simulink model "TrafficLightNegotiationWithV2XTestBench"  (R2024b)
settings: Solver=ode23tb  StartTime=0.0  StopTime=scenario.StopTime  FixedStep=0.1  RelTol=1e-8  EnableMultiTasking=on
PostLoadFcn:
  | helperSLTrafficLightNegotiationWithV2XSetup
values from neighbouring files (symbols this model uses):
  actorsClassID = [[profiles.ActorID]' [profiles.ClassID]' [profiles.Length]' [profiles.Width]']    [helperSLTrafficLightNegotiationWithV2XSetup.m]
  intersectionInfo = evalin('base', 'intersectionInfo')    [HelperTLNwithV2XVisualization.m]
  posSelector = [ 1, 0, 0, 0, 0, 0, 0, 0, 0; 0, 0, 0, 1, 0, 0, 0, 0, 0]    [helperSLTrafficLightNegotiationWithV2XSetup.m]
  referencePathInfo = helperEgoRefPathCreator(scenario, egoVehicle.ActorID)    [helperSLTrafficLightNegotiationWithV2XSetup.m]
  sceneOrigin = [42.2995, -83.6990, 0]    [helperSLTrafficLightNegotiationWithV2XSetup.m]
undefined symbols (not defined in the file or in its folder): M, N, Ts, v_set
libraries: drivingscenarioandsensors x2, simulink x1, drivinglib x1
CloseFcn:
  | helperSLTrafficLightNegotiationWithV2XCleanUp
settings Model: SnapshotBufferSize=50  SnapshotInterval=1  Creator=The MathWorks, Inc.  LastModifiedBy=Pranith
settings SolverCC: ZeroCrossAlgorithm=Adaptive  AlgebraicLoopSolver=TrustRegion  PositivePriorityOrder=on  AutoInsertRateTranBlk=on  InsertRTBMode=Always  DecoupledContinuousIntegration=on  MinimalZcImpactIntegration=on  MaxZcPerStep=1
settings DataIOCC: SaveOutput=off  SaveTime=off  ReturnWorkspaceOutputs=off
settings OptimizationCC: ReuseModelBlockBuffer=off
settings DebuggingCC: MaskedZcDiagnostic=none  IgnoredZcDiagnostic=none  ParameterPrecisionLossMsg=none  UnconnectedInputMsg=warning  UnconnectedOutputMsg=warning  UnconnectedLineMsg=warning  PregeneratedLibrarySubsystemCodeDiagnostic=none  SubsystemReferenceDiagnosticForUnitTest=warning  ArithmeticOperatorsInVariantConditions=warning
settings HardwareCC: ProdLongLongMode=on
settings ModelReferenceCC: EnableRefExpFcnMdlSchedulingChecks=on
settings SFSimCC: SimUseLocalCustomCode=off
settings RTWCC: GenerateReport=on  RTWUseLocalCustomCode=off  LaunchReport=on  GPUComputeCapability=3.5  DLArmComputeVersion=19.05
settings ConfigComp: CovScope=ReferencedModels  CovIncludeTopModel=off

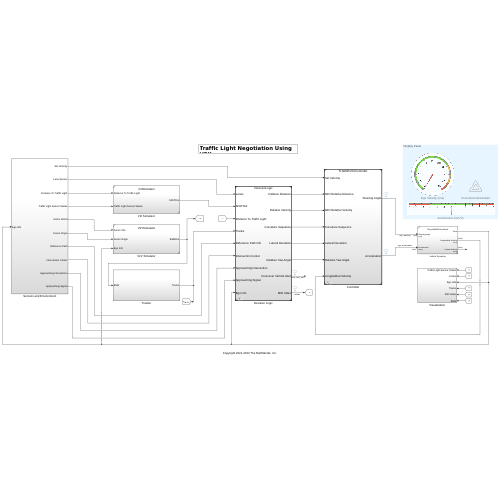
[thumbnail: Simulink's stored preview of the top-level diagram]
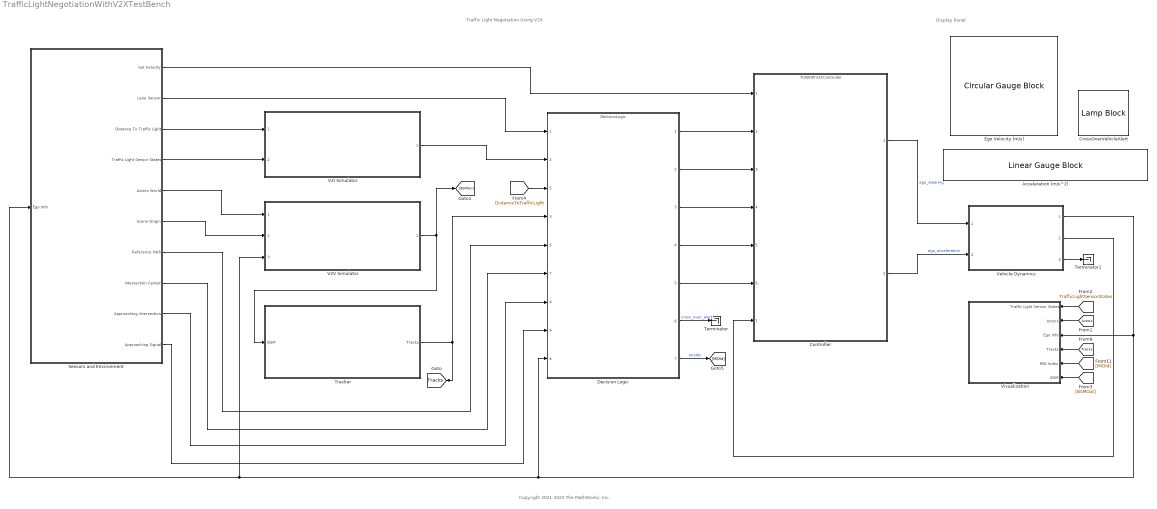
== system TrafficLightNegotiationWithV2XTestBench ==
  note: Traffic Light Negotiation Using V2X
  note: Display Panel
  note: Copyright 2021-2023 The MathWorks, Inc.
  Acceleration (m/s^2) : LinearGaugeBlock  LabelPosition=Hide  ScaleMin=-6  ScaleMax=6
  Controller : ModelReference  ModelNameDialog=TLNWithV2XController.slx  SimulationMode=Normal  ModelReferenceVersion=5.0
  CrossOverVehicleAlert : LampBlock  LabelPosition=Hide  Icon=Hazards
  Decision Logic : ModelReference  ModelNameDialog=DecisionLogic.slx  SimulationMode=Normal  ModelReferenceVersion=9.1
      settings: PortSchema="{\"entries\":[{\"content\":{\"sides\":[{\"content\":{\"connectorIds\":[\"In1\",\"In2\",\"In5\",\"In3\",\"In6\",\"In7\",\"In8\",\"In9\",\"In4\"]},\"type\":\"ConnectorPlacement.EquallySpacedRectSide\",\"uuid\":\"580d7771-a392-489d-ba06-e0a23417c921\"},{\"content\":{\"connectorIds\":[\"Out1\",\"Out2\",\"Out3\",\"Out4\",\"Out5\",\"Out6\",\"Out7\"],\"side\":\"RIGHT\"},\"type\":\"ConnectorPlacement.EquallySpacedRectSide\",\"uuid\":\"34dc41bc-0d5b-42f7-ac4d-a18cefff1604\"},{\"content\":{\"connectorIds\":[],\"side\":\"TOP\"},\"type\":\"ConnectorPlacement.EquallySpacedRectSide\",\"uuid\":\"c461dccf-2cc6-49a6-b643-9bb66a30f56a\"},{\"content\":{\"connectorIds\":[],\"side\":\"HIDDEN\"},\"type\":\"ConnectorPlacement.EquallySpacedRectSide\",\"uuid\":\"944284c5-f0c1-462b-8985-62524d7ec2e9\"}]},\"type\":\"ConnectorPlacement.EquallySpacedConnector\",\"uuid\":\"d6b87f41-7423-4eb9-8350-a9de1b3f3f98\"}],\"packageUris\":[\"http://schema.mathworks.com/mf0/Connector/R2020b\"],\"version\":\"1.0\"}"
  Ego Velocity (m/s) : CircularGaugeBlock  LabelPosition=Hide  ScaleMax=50
  Sensors and Environment : Subsystem
  Terminator : Terminator
  Terminator1 : Terminator
  Tracker : Subsystem
  V2I Simulator : Subsystem  ReferencedSubsystem=V2ISimulator
  V2V Simulator : Subsystem  ReferencedSubsystem=V2VSimulator
  Vehicle Dynamics : Subsystem  ReferencedSubsystem=BicycleWithForceInput
  Visualization : Subsystem
  tag scope: Tracks=global
  wires:
  [TrafficLightSensorStates] -> Visualization/1(Traffic Light Sensor States)
  Vehicle Dynamics/1 -> V2V Simulator/3, Sensors and Environment/1(Ego Info), Decision Logic/4, Visualization/3(Ego Info)
  [Actors] -> Visualization/2(Actors)
  [Tracks] -> Visualization/4(Tracks)
  [MIOId] -> Visualization/5(MIO Index)
  Decision Logic/6 -> Terminator/1  "cross_over_alert"
  [DistanceToTrafficLight] -> Decision Logic/5
  Sensors and Environment/2(Lane Sensor) -> Decision Logic/1
  V2I Simulator/1 -> Decision Logic/2
  V2V Simulator/1 -> [BSMOut], Tracker/1(BSM)
  Tracker/1(Tracks) -> Decision Logic/3, [Tracks]
  Vehicle Dynamics/3 -> Terminator1/1
  [BSMOut] -> Visualization/6(BSM)
  Sensors and Environment/3(Distance To Traffic Light) -> V2I Simulator/1
  Sensors and Environment/4(Traffic Light Sensor States) -> V2I Simulator/2
  Sensors and Environment/5(Actors World) -> V2V Simulator/1
  Sensors and Environment/6(Scene Origin) -> V2V Simulator/2
  Sensors and Environment/10(Approaching Signal) -> Decision Logic/9
  Sensors and Environment/9(Approaching Intersection) -> Decision Logic/8
  Sensors and Environment/8(Intersection Center) -> Decision Logic/7
  Sensors and Environment/7(Reference Path) -> Decision Logic/6
  Decision Logic/7 -> [MIOId]  "mioIdx"
  Sensors and Environment/1(Set Velocity) -> Controller/1
  Decision Logic/5 -> Controller/6
  Decision Logic/4 -> Controller/5
  Decision Logic/3 -> Controller/4
  Decision Logic/2 -> Controller/3
  Decision Logic/1 -> Controller/2
  Controller/1 -> Vehicle Dynamics/1  "ego_steering"
  Controller/2 -> Vehicle Dynamics/2  "ego_acceleration"
  Vehicle Dynamics/2 -> Controller/7

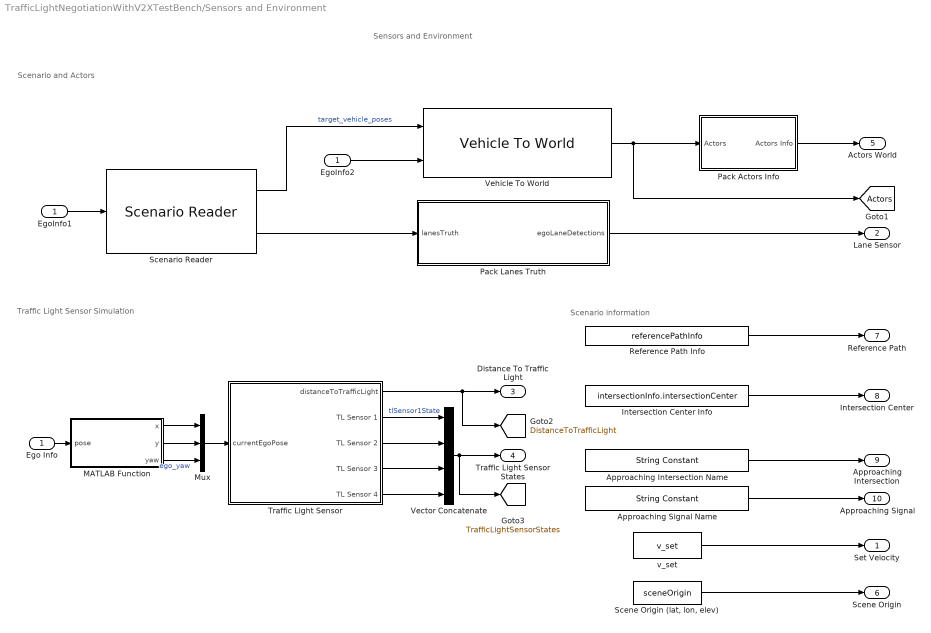
== system TrafficLightNegotiationWithV2XTestBench/Sensors and Environment ==
  note: Scenario information
  note: Traffic Light Sensor Simulation
  note: Scenario and Actors
  note: Sensors and Environment
  Ego Info : Inport
  Approaching Intersection Name : StringConstant  String=approachingIntersectionName
  Approaching Signal Name : StringConstant  String=approachingSignalName
  EgoInfo1 : InportShadow
  EgoInfo2 : InportShadow
  Intersection Center Info : Constant  Value=intersectionInfo.intersectionCenter  SampleTime=Ts
      settings: AttributesFormatString=|
      | ------------------------------
      |    Value = %<Value>
  MATLAB Function : MATLAB Function  TreatAsAtomicUnit=on
  Mux : Mux  Inputs=3
  Pack Actors Info : Subsystem
  Pack Lanes Truth : MATLAB Function  TreatAsAtomicUnit=on  mask{detStructObj=Simulink.Bus.createMATLABStruct('LaneSensor')}
      mask prompts: detStructObj "Output lane detections struct"
  Reference Path Info : Constant  Value=referencePathInfo  OutDataTypeStr=Bus: ReferencePathInfo  SampleTime=Ts
      settings: AttributesFormatString=|
      | --------------------------
      |   Value = %<Value>
  Scenario Reader : drivingscenarioandsensors/Scenario Reader  ScenarioSource=From workspace  ScenarioFileName=C:\Users\rsuresh\OneDrive - MathWorks\Desktop\V2X\V2X_DesignReview_V1.2\MultiVehicleScenario.mat  ScenarioVariableName=scenario  OutputCoordinateSystem=Vehicle coordinates  EgoVehicleSource=Input port  EgoVehicleActorID=egoVehicle.ActorID  OrientVehiclesOnRoad=on  OutputEgoVehiclePose=off  OutputEgoVehicleState=off  SampleTime=Ts  LaneBoundaryOutput=Ego vehicle lane boundaries  LaneBoundaryDistance=0:0.5:9.5  LaneBoundaryLocation=Center of lane markings  BusNameSource=Property  BusName=BusActors  BusNumActorsSource=Property  BusNumActors=12  BusName2Source=Property  BusName2=BusLaneBoundaries  BusNumLaneBoundariesSource=Scenario  BusNumLaneBoundaries=10  BusName3Source=Auto  BusName3=BusEgoActor  BusName4Source=Auto  BusName4=BusEgoState  ShowCoordinateLabels=on  SimulateUsing=Interpreted execution
  "Scene Origin (lat, lon, elev)" : Constant  Value=sceneOrigin  SampleTime=Ts
  Traffic Light Sensor : Subsystem  mask{TrafficLightSensorModeSelection=Cycle, TrafficLightPosition=intersectionInfo.tlSensor1Position}
      mask prompts: TrafficLightSensorModeSelection "Traffic Light Sensor Mode:"; TrafficLightPosition "Traffic Light Position:"
      mask TypeOptions TrafficLightSensorModeSelection: Steady Green | Steady Red | Cycle
      mask TypeOptions TrafficLightPosition: TrafficLightPosition/Value
      mask DialogControl DescTextVar Prompt: Simulate a traffic light sensor.
  Vector Concatenate : Concatenate  NumInputs=4  Mode=Multidimensional array
  Vehicle To World : drivingscenarioandsensors/Vehicle To World  BusNameSource=Property  BusName=BusVehicleToWorldActors  SimulateUsing=Interpreted execution
  v_set : Constant  Value=v_set  SampleTime=Ts
  Set Velocity : Outport
  Lane Sensor : Outport  Port=2  VectorParamsAs1DForOutWhenUnconnected=off
  Distance To Traffic Light : Outport  Port=3
  Traffic Light Sensor States : Outport  Port=4
  Actors World : Outport  Port=5  OutDataTypeStr=Bus: BusActorsInfo
  Scene Origin : Outport  Port=6
  Reference Path : Outport  Port=7
  Intersection Center : Outport  Port=8
  Approaching Intersection : Outport  Port=9  OutDataTypeStr=string
  Approaching Signal : Outport  Port=10  OutDataTypeStr=string
  tag scope: Actors=global, DistanceToTrafficLight=global, TrafficLightSensorStates=global
  wires:
  Ego Info/1 -> MATLAB Function/1(pose)
  MATLAB Function/3(yaw) -> Mux/3  "ego_yaw"
  MATLAB Function/2(y) -> Mux/2
  MATLAB Function/1(x) -> Mux/1
  Mux/1 -> Traffic Light Sensor/1(currentEgoPose)
  Scenario Reader/1 -> Vehicle To World/1  "target_vehicle_poses"
  EgoInfo1/1 -> Scenario Reader/1
  Reference Path Info/1 -> Reference Path/1
  v_set/1 -> Set Velocity/1
  Intersection Center Info/1 -> Intersection Center/1
  Traffic Light Sensor/2(TL Sensor 1) -> Vector Concatenate/1  "tlSensor1State"
  Traffic Light Sensor/3(TL Sensor 2) -> Vector Concatenate/2
  Traffic Light Sensor/4(TL Sensor 3) -> Vector Concatenate/3
  Traffic Light Sensor/5(TL Sensor 4) -> Vector Concatenate/4
  EgoInfo2/1 -> Vehicle To World/2
  Vehicle To World/1 -> Pack Actors Info/1(Actors), [Actors]
  Vector Concatenate/1 -> Traffic Light Sensor States/1, [TrafficLightSensorStates]
  "Scene Origin (lat, lon, elev)"/1 -> Scene Origin/1
  Traffic Light Sensor/1(distanceToTrafficLight) -> [DistanceToTrafficLight], Distance To Traffic Light/1
  Pack Lanes Truth/1(egoLaneDetections) -> Lane Sensor/1
  Scenario Reader/2 -> Pack Lanes Truth/1(lanesTruth)
  Approaching Signal Name/1 -> Approaching Signal/1
  Approaching Intersection Name/1 -> Approaching Intersection/1
  Pack Actors Info/1(Actors Info) -> Actors World/1

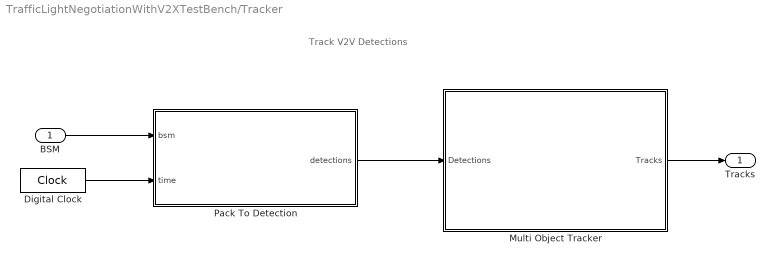
== system TrafficLightNegotiationWithV2XTestBench/Tracker ==
  note: Track V2V Detections
  BSM : Inport  OutDataTypeStr=Bus: BusBSM  SampleTime=Ts
  Digital Clock : DigitalClock  SampleTime=Ts
  Multi Object Tracker : Subsystem
  Pack To Detection : MATLAB Function  TreatAsAtomicUnit=on  mask{origin=sceneOrigin, outputStruct=Simulink.Bus.createMATLABStruct('BusTargetDetections')}
      mask prompts: origin "Scene Origin"; outputStruct "Output Struct"
  Tracks : Outport
  wires:
  BSM/1 -> Pack To Detection/1(bsm)
  Pack To Detection/1(detections) -> Multi Object Tracker/1(Detections)
  Multi Object Tracker/1(Tracks) -> Tracks/1
  Digital Clock/1 -> Pack To Detection/2(time)

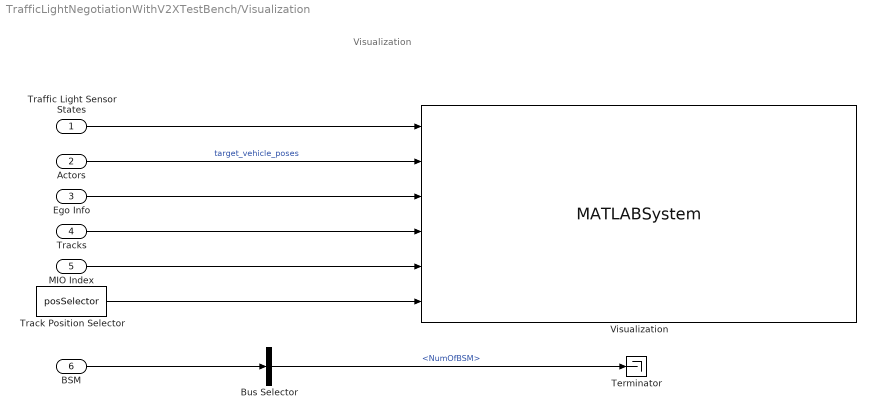
== system TrafficLightNegotiationWithV2XTestBench/Visualization ==
  note: Visualization
  Traffic Light Sensor States : Inport
  Actors : Inport  Port=2
  Ego Info : Inport  Port=3
  Tracks : Inport  Port=4
  MIO Index : Inport  Port=5
  BSM : Inport  Port=6
  Bus Selector : BusSelector  OutputSignals=NumOfBSM
  Terminator : Terminator
  Track Position Selector : Constant  Value=posSelector
  Visualization : MATLABSystem  System=HelperTLNwithV2XVisualization  range=V2XRange  TrafficLightDisp=on  EnableVisualization=on
      mask Type: HelperTLNwithV2XVisualization
      mask Display:
      | disp('HelperTLNwithV2XVisualization');
      | port_label('input',1,'trafficLightSensorStates');
      | port_label('input',2,'targetPoses');
      | port_label('input',3,'egoInfo');
      | port_label('input',4,'tracks');
      | port_label('input',5,'mioIndex');
      | port_label('input',6,'posSelector');
  wires:
  Traffic Light Sensor States/1 -> Visualization/1
  Ego Info/1 -> Visualization/3
  Actors/1 -> Visualization/2  "target_vehicle_poses"
  Tracks/1 -> Visualization/4
  MIO Index/1 -> Visualization/5
  Track Position Selector/1 -> Visualization/6
  BSM/1 -> Bus Selector/1
  Bus Selector/1 -> Terminator/1  "<NumOfBSM>"

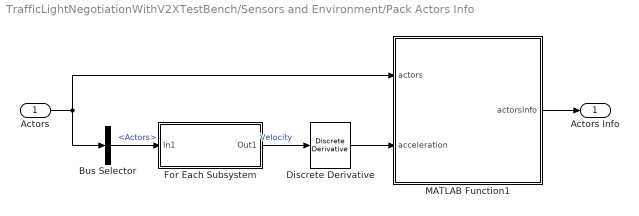
== system TrafficLightNegotiationWithV2XTestBench/Sensors and Environment/Pack Actors Info ==
  Actors : Inport
  Bus Selector : BusSelector  OutputSignals=Actors
  Discrete Derivative : simulink/Discrete/Discrete Derivative  gainval=1.0  ICPrevScaledInput=0.0  OutMin=[]  OutMax=[]  OutDataType=fixdt(1, 16)  OutScaling=2^-10  DoSatur=off
  For Each Subsystem : Subsystem  TreatAsAtomicUnit=on
  MATLAB Function1 : MATLAB Function  TreatAsAtomicUnit=on  mask{outputStruct=Simulink.Bus.createMATLABStruct('BusActorsInfo')}
      mask prompts: outputStruct "Output Struct"
  Actors Info : Outport
  wires:
  MATLAB Function1/1(actorsInfo) -> Actors Info/1
  Actors/1 -> Bus Selector/1, MATLAB Function1/1(actors)
  Bus Selector/1 -> For Each Subsystem/1(In1)  "<Actors>"
  For Each Subsystem/1(Out1) -> Discrete Derivative/1  "Velocity"
  Discrete Derivative/1 -> MATLAB Function1/2(acceleration)

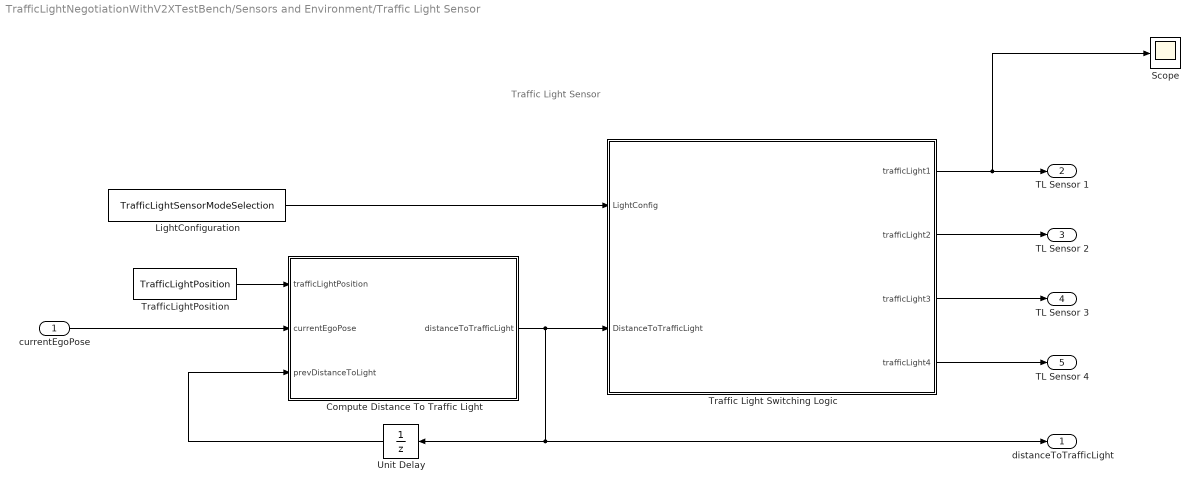
== system TrafficLightNegotiationWithV2XTestBench/Sensors and Environment/Traffic Light Sensor ==
  note: Traffic Light Sensor
  currentEgoPose : Inport
  Compute Distance To Traffic Light : MATLAB Function  TreatAsAtomicUnit=on  mask{minTLDist=3}
      mask prompts: minTLDist "Minimum distance to traffic light"
  LightConfiguration : Constant  Value=TrafficLightSensorModeSelection
  Scope : Scope
  Traffic Light Switching Logic : Stateflow chart  TreatAsAtomicUnit=on
      settings: PortSchema="{\"entries\":[{\"content\":{\"sides\":[{\"content\":{\"connectorIds\":[\"In2\",\"In1\"]},\"type\":\"ConnectorPlacement.EquallySpacedRectSide\",\"uuid\":\"7756c064-2a7e-4f45-95ae-d682ad49d06b\"},{\"content\":{\"connectorIds\":[\"Out1\",\"Out2\",\"Out3\",\"Out4\"],\"side\":\"RIGHT\"},\"type\":\"ConnectorPlacement.EquallySpacedRectSide\",\"uuid\":\"6c34b4bd-9c36-46df-bdd3-7c2894bd4199\"},{\"content\":{\"connectorIds\":[],\"side\":\"TOP\"},\"type\":\"ConnectorPlacement.EquallySpacedRectSide\",\"uuid\":\"fd108523-5003-412a-b183-16db0b55cab1\"}]},\"type\":\"ConnectorPlacement.EquallySpacedConnector\",\"uuid\":\"244779f5-6045-4784-a339-0cb30d4bfa7f\"}],\"packageUris\":[\"http://schema.mathworks.com/mf0/Connector/19700101\"],\"version\":\"1.0\"}"
  TrafficLightPosition : Constant  Value=TrafficLightPosition
  Unit Delay : UnitDelay  InitialCondition=100  SampleTime=-1  HasFrameUpgradeWarning=on
  distanceToTrafficLight : Outport
  TL Sensor 1 : Outport  Port=2  PortDimensions=1
  TL Sensor 2 : Outport  Port=3  PortDimensions=1
  TL Sensor 3 : Outport  Port=4  PortDimensions=1
  TL Sensor 4 : Outport  Port=5  PortDimensions=1
  wires:
  TrafficLightPosition/1 -> Compute Distance To Traffic Light/1(trafficLightPosition)
  Unit Delay/1 -> Compute Distance To Traffic Light/3(prevDistanceToLight)
  currentEgoPose/1 -> Compute Distance To Traffic Light/2(currentEgoPose)
  LightConfiguration/1 -> Traffic Light Switching Logic/2(LightConfig)
  Traffic Light Switching Logic/1(trafficLight1) -> Scope/1, TL Sensor 1/1
  Traffic Light Switching Logic/4(trafficLight4) -> TL Sensor 4/1
  Traffic Light Switching Logic/3(trafficLight3) -> TL Sensor 3/1
  Traffic Light Switching Logic/2(trafficLight2) -> TL Sensor 2/1
  Compute Distance To Traffic Light/1(distanceToTrafficLight) -> distanceToTrafficLight/1, Unit Delay/1, Traffic Light Switching Logic/1(DistanceToTrafficLight)

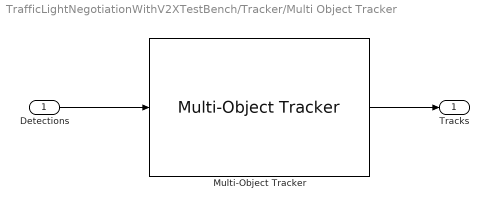
== system TrafficLightNegotiationWithV2XTestBench/Tracker/Multi Object Tracker ==
  Detections : Inport  OutDataTypeStr=Bus: BusTargetDetections
  Multi-Object Tracker : drivinglib/Multi-Object Tracker  TrackerIndex=uint32( 0 )  FilterInitializationFcn=initcaekf  AssignmentThreshold=assignThresh  ConfirmationThreshold=[M N]  DeletionThreshold=[ 5, 5 ]  MaxNumTracks=numTracks  MaxNumSensors=numSensors  OOSMHandling=Terminate  StateParametersSimulink=struct  HasStateParametersInput=off  TimeInputSource=Auto  HasCostMatrixInput=off  HasDetectableTrackIDsInput=off  BusNameSource=Property  BusName=BusMultiObjectTracker  TentativeTracksOutputPort=off  AllTracksOutputPort=off  SimulateUsing=Interpreted execution
  Tracks : Outport
  wires:
  Multi-Object Tracker/1 -> Tracks/1
  Detections/1 -> Multi-Object Tracker/1

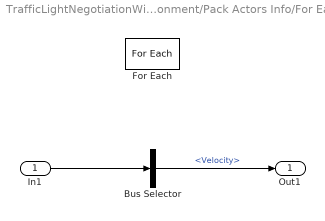
== system TrafficLightNegotiationWithV2XTestBench/Sensors and Environment/Pack Actors Info/For Each Subsystem ==
  In1 : Inport  Partition=on  PartitionDimension=1  PartitionWidth=1  PartitionOffset=0
  Bus Selector : BusSelector  OutputSignals=Velocity
  For Each : ForEach  DisableCoverage=on
  Out1 : Outport  ConcatenationDimension=1
  wires:
  In1/1 -> Bus Selector/1
  Bus Selector/1 -> Out1/1  "<Velocity>"

== matlab function TrafficLightNegotiationWithV2XTestBench/Sensors and Environment/Pack Lanes Truth ==
  data: egoLaneDetections output Bus: LaneSensor; lanesTruth input; detStructObj parameter
function egoLaneDetections = packLanesTruth(lanesTruth, detStructObj)
% Assign lane parameters from ground-truth lane boundaries.

% Assign lane detections struct object to output variable
egoLaneDetections = detStructObj;

% Find ego-vehicle lane boundary indices
lbNum = [1, 1];
for j = 1:length(lanesTruth.LaneBoundaries)-1
    yleftLane = lanesTruth.LaneBoundaries(j+1).Coordinates(1,2);
    yrightLane = lanesTruth.LaneBoundaries(j).Coordinates(1,2);
    
    if ((0 >= yleftLane) && (0 <= yrightLane))
        lbNum(1) = j;
        lbNum(2) = j+1;
        break;
    elseif ((0 >= yrightLane) && (0 <= yleftLane))
        lbNum(1) = j+1;
        lbNum(2) = j;
        break;
    end
end

%% Pack left lane info
coder.varsize('leftLaneCoordinates')
leftLaneCoordinates = lanesTruth.LaneBoundaries(lbNum(1)).Coordinates;
idx = ~isfinite(leftLaneCoordinates(:,1));
leftLaneCoordinates(idx,:) = [];
if size(leftLaneCoordinates,1) > 2
    % Get parabolic lane boundary parameters using polyfit for the left lane.
    leftLaneParameters = polyfit(leftLaneCoordinates(:,1),...
        leftLaneCoordinates(:,2),2);
    
    % Assign left lane parameters to output bus, lanes.
    egoLaneDetections.Left.Curvature = single(2 * leftLaneParameters(1));
    egoLaneDetections.Left.HeadingAngle = single(leftLaneParameters(2));
    egoLaneDetections.Left.LateralOffset = single(leftLaneParameters(3));
    
    egoLaneDetections.Left.Strength = single(lanesTruth.LaneBoundaries(lbNum(1)).Strength);
end


%% Pack right lane info
coder.varsize('rightLaneCoordinates')
rightLaneCoordinates = lanesTruth.LaneBoundaries(lbNum(2)).Coordinates;
idx = ~isfinite(rightLaneCoordinates(:,1));
rightLaneCoordinates(idx,:) = [];
if size(rightLaneCoordinates,1) > 2
    % Get parabolic lane boundary parameters using polyfit for the right lane
    rightLaneParameters = polyfit(rightLaneCoordinates(:,1),...
        rightLaneCoordinates(:,2),2);
    
    % Assign right lane parameters to output bus, lanes.
    egoLaneDetections.Right.Curvature = single(2 * rightLaneParameters(1));
    egoLaneDetections.Right.HeadingAngle = single(rightLaneParameters(2));
    egoLaneDetections.Right.LateralOffset = single(rightLaneParameters(3));
    
    egoLaneDetections.Right.Strength = single(lanesTruth.LaneBoundaries(lbNum(2)).Strength);
end
end

== matlab function TrafficLightNegotiationWithV2XTestBench/Sensors and Environment/Pack Actors Info/MATLAB Function1 ==
  data: actors input; acceleration input; actorsInfo output Bus: BusActorsInfo; actorsClassID parameter; outputStruct parameter
function actorsInfo = addActorProfiles(actors,acceleration,actorsClassID,outputStruct) 
    actorsInfo = outputStruct;
    outputStruct.NumActors = actors.NumActors;
    outputStruct.Time      = actors.Time;
    for i = 1:actors.NumActors
        outputStruct.Actors(i).ActorID  = actors.Actors(i).ActorID;
        classId = actorsClassID((actorsClassID(:,1) == actors.Actors(i).ActorID) ,2);
        length  = actorsClassID((actorsClassID(:,1) == actors.Actors(i).ActorID) ,3);
        width   = actorsClassID((actorsClassID(:,1) == actors.Actors(i).ActorID) ,4);
        outputStruct.Actors(i).ClassID  = classId(1);
        outputStruct.Actors(i).Position = actors.Actors(i).Position;
        outputStruct.Actors(i).Velocity = actors.Actors(i).Velocity;
        outputStruct.Actors(i).Acceleration = acceleration(i,:);
        outputStruct.Actors(i).Roll  = actors.Actors(i).Roll;
        outputStruct.Actors(i).Pitch = actors.Actors(i).Pitch;
        outputStruct.Actors(i).Yaw   = actors.Actors(i).Yaw;
        outputStruct.Actors(i).Length   = length(1);
        outputStruct.Actors(i).Width   = width(1);
    end
    actorsInfo = outputStruct;
end

== matlab function TrafficLightNegotiationWithV2XTestBench/Sensors and Environment/Traffic Light Sensor/Compute Distance To Traffic Light ==
  data: trafficLightPosition input; currentEgoPose input; prevDistanceToLight input; distanceToTrafficLight output; minTLDist parameter
function distanceToTrafficLight   = computeDistanceToTrafficLight(trafficLightPosition, currentEgoPose, prevDistanceToLight, minTLDist)
    % helperComputeDistanceToTrafficLight Compute distance to upcoming traffic
    % light.
    %
    % Current Ego position and the upcoming traffic light position information
    % are used for calculating distance to traffic light. 
    %
    % NOTE: This is a helper function for example purposes and may be removed or
    % modified in the future.
    %
    
    % Copyright 2021 The MathWorks, Inc.
    
    % Once the vehicle reaches the traffic light, it should see the next
    % traffic light if any. In this example, there is no next traffic light so
    % the next traffic light is assumed at infinite distance. 
    %
    % if the previous distance between the vehicle and the traffic light is
    % less than the minTLDist, then it is treated that vehicle has passed the
    % light.
    
    if(prevDistanceToLight < minTLDist || prevDistanceToLight == Inf)
        distanceToTrafficLight = inf;
    else
        % Euclidean distance to upcoming traffic light from the current
        % position of ego vehicle.
        %
        distanceToTrafficLight = double(sqrt((trafficLightPosition(1)-currentEgoPose(1))^2 + ...
            (trafficLightPosition(2)-currentEgoPose(2))^2));
    end
end

== matlab function TrafficLightNegotiationWithV2XTestBench/Tracker/Pack To Detection ==
  data: bsm input Bus: BusBSM; detections output Bus: BusTargetDetections; origin parameter; outputStruct parameter; time input
function detections = packToDetection(bsm,origin, outputStruct, time)

detections = outputStruct; 
if bsm.NumOfBSM>0
    detections.NumDetections = bsm.NumOfBSM;
    measCov = cast(diag([1,1,1,1,1,1]),'double');
    measparms = struct('Frame',drivingCoordinateFrameType(1),...
        'OriginPosition',zeros(3,1,'double'),...
        'Orientation',eye(3,'double'),...
        'HasVelocity',true, ...
        'HasElevation',false);

    for idx = 1:bsm.NumOfBSM        
        BSMCoreData = bsm.BSMCoreData(idx);
        
        lla = [double(BSMCoreData.Lattitude)*10^-7,...
            double(BSMCoreData.Longitude)*10^-7,...
            double(BSMCoreData.Elevation)*0.1];
        
        % Transform geodetic coordinates to local east-north-up coordinates

        pos = [0 0 0];
        [pos(1),pos(2),pos(3)] = latlon2local(lla(1),lla(2),lla(3),origin);
        speed = double(BSMCoreData.Speed)*0.02;
        heading = double(BSMCoreData.Heading)*0.0125;
        vy = speed*cosd(heading);
        vx = speed*sind(heading);
        
        detections.Detections(idx).Time = time;double(BSMCoreData.SecMark)*1e-3;
        detections.Detections(idx).Measurement = [pos(1); pos(2); 0; vx; vy; 0]; % [x;y;z;vx;vy;vz]
        detections.Detections(idx).MeasurementNoise = measCov;
        detections.Detections(idx).SensorIndex = 1;
        detections.Detections(idx).ObjectClassID = 1;
        detections.Detections(idx).MeasurementParameters = measparms;
    end
end

end

== matlab function TrafficLightNegotiationWithV2XTestBench/Sensors and Environment/MATLAB Function ==
  data: pose input; x output; y output; yaw output
function [x, y, yaw] = poseToSim(pose)

pos_Rr = pose.Position([1,2])';
theta = pose.Yaw;

pos_Cen = pos_Rr+[cosd(theta) sind(theta)]';

x = pos_Cen(1);
y = pos_Cen(2);
yaw = pose.Yaw;

== stateflow chart TrafficLightNegotiationWithV2XTestBench/Sensors and Environment/Traffic Light Sensor/Traffic Light Switching Logic ==
  state STEADYRED
    entry:
    trafficLight1 = Red;
    trafficLight2 = Green;
    trafficLight3 = Red;
    trafficLight4 = Green;
  state START
    entry:
    trafficLight1 = Red;
    trafficLight2 = Red;
    trafficLight3 = Red;
    trafficLight4 = Red;
  state STEADYGREEN
    entry:
    trafficLight1 = Green;
    trafficLight2 = Red;
    trafficLight3 = Green;
    trafficLight4 = Red;
  state TRAFFICLIGHT1GREEN
    entry:
    trafficLight1 = Green;
    trafficLight2 = Red;
    trafficLight3 = Green;
    trafficLight4 = Red;
  state TRAFFICLIGHT1YELLOW
    entry:
    trafficLight1 = Yellow;
    trafficLight2 = Red;
    trafficLight3 = Yellow;
    trafficLight4 = Red;
  state TRAFFICLIGHT2GREEN
    entry:
    trafficLight1 = Red;
    trafficLight2 = Green;
    trafficLight3 = Red;
    trafficLight4 = Green;
  state TRAFFICLIGHT2YELLOW
    entry:
    trafficLight1 = Red;
    trafficLight2 = Yellow;
    trafficLight3 = Red;
    trafficLight4 = Yellow;
  (default) -> START
  START -> STEADYRED [order 2] : [DistanceToTrafficLight < trafficLightStateTriggerThreshold ...
      | && LightConfig==2]
  START -> STEADYGREEN [order 3] : [DistanceToTrafficLight < trafficLightStateTriggerThreshold ...
      |  && LightConfig==1]
  START -> TRAFFICLIGHT1GREEN [order 1] : [DistanceToTrafficLight < trafficLightStateTriggerThreshold && LightConfig ==3]
  TRAFFICLIGHT1GREEN -> TRAFFICLIGHT1YELLOW : after(4.2,sec)
  TRAFFICLIGHT2YELLOW -> TRAFFICLIGHT1GREEN : after(0.5,sec)
  TRAFFICLIGHT1YELLOW -> TRAFFICLIGHT2GREEN : after(0.5,sec)
  TRAFFICLIGHT2GREEN -> TRAFFICLIGHT2YELLOW : after(4,sec)
  data: trafficLight1 output; trafficLight2 output; trafficLight3 output; trafficLight4 output; Green constant double =2; Red constant double =0; Yellow constant double =1; DistanceToTrafficLight input; trafficLightStateTriggerThreshold parameter; LightConfig input
